simulink model "Exp_3_batch_17_Simulation (2)"  (R2020a)
settings: Solver=VariableStepAuto  StartTime=0.0  StopTime=20  RelTol=1e-3
settings Model: Creator=sundaram bhupathi  LastModifiedBy=tarun

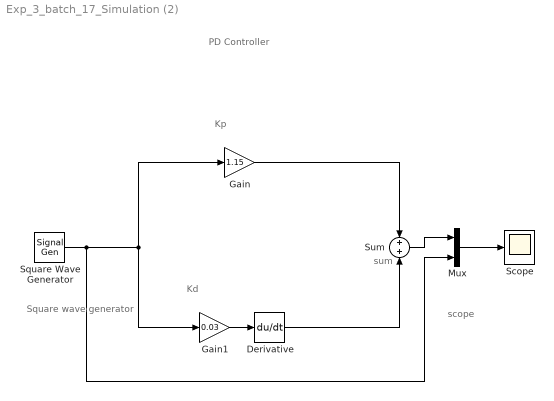
== system Exp_3_batch_17_Simulation (2) ==
  note: Kd
  note: Kp
  note: PD Controller
  note: scope
  note: Square wave generator
  note: sum
  Derivative : Derivative
  Gain : Gain  Gain=1.15
  Gain1 : Gain  Gain=0.03
  Mux : Mux  Inputs=2
  Scope : Scope
  Square Wave Generator : SignalGenerator  WaveForm=square  Amplitude=10  Units=rad/sec
  Sum : Sum  InputSameDT=on  SaturateOnIntegerOverflow=on  OutDataTypeStr=Inherit: Same as first input
  wires:
  Derivative/1 -> Sum/2
  Gain/1 -> Sum/1
  Sum/1 -> Mux/1
  Gain1/1 -> Derivative/1
  Square Wave Generator/1 -> Mux/2, Gain1/1, Gain/1
  Mux/1 -> Scope/1
